simulink subsystem "PID_nadir"  (R2021a)
settings: Solver=VariableStepAuto  StartTime=0.0  StopTime=10.0  RelTol=1e-3
undefined symbols (not defined in the file): Max_magmom, Min_magmom
libraries: sharedutil x1
settings Model: Creator=Laura  LastModifiedBy=Laura

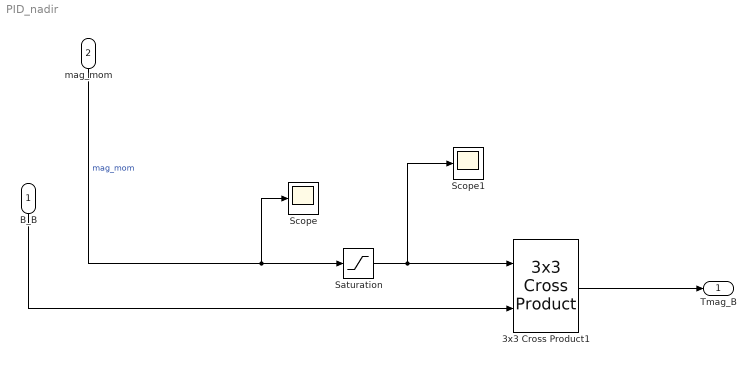
== system PID_nadir ==
  B_B : Inport
  mag_mom : Inport  Port=2
  3x3 Cross Product1 : sharedutil/3x3 Cross Product  aMode=aMode
      settings: SourceProductBaseCode=AE,PW,DR,MT,UV,VE
  Saturation : Saturate  UpperLimit=Max_magmom  LowerLimit=Min_magmom
  Scope : Scope
  Scope1 : Scope
  Tmag_B : Outport
  wires:
  B_B/1 -> 3x3 Cross Product1/2
  mag_mom/1 -> Scope/1, Saturation/1  "mag_mom"
  3x3 Cross Product1/1 -> Tmag_B/1
  Saturation/1 -> 3x3 Cross Product1/1, Scope1/1
